simulink model "motion_planner"  (R2015a)
settings: Solver=ode45  StartTime=0.0  StopTime=10.0  RelTol=1e-3
libraries: robotlib x9
settings Model: Creator=Kelan  LastModifiedBy=Kelan

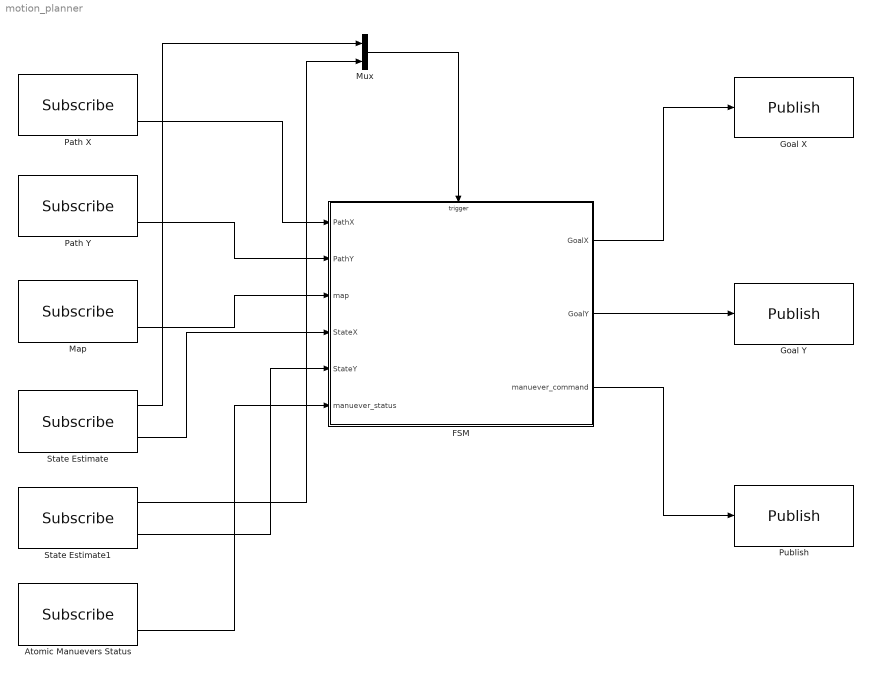
== system motion_planner ==
  Atomic Manuevers Status : robotlib/Subscribe  SourceLibraryInfo=This block requires Robotics System Toolbox  topicSource=Specify your own  topic=/manuevers_status  messageType=std_msgs/Bool  sampleTime=-1  messageQueueLength=1
  FSM : Stateflow chart  TreatAsAtomicUnit=on
  Goal X : robotlib/Publish  SourceLibraryInfo=This block requires Robotics System Toolbox  topicSource=Specify your own  topic=/GoalX  messageType=std_msgs/Int16  messageQueueLength=1
  Goal Y : robotlib/Publish  SourceLibraryInfo=This block requires Robotics System Toolbox  topicSource=Specify your own  topic=/GoalY  messageType=std_msgs/Int16  messageQueueLength=1
  Map : robotlib/Subscribe  SourceLibraryInfo=This block requires Robotics System Toolbox  topicSource=Specify your own  topic=/map  messageType=nav_msgs/OccupancyGrid  sampleTime=-1  messageQueueLength=1
  Mux : Mux  Inputs=2
  Path X : robotlib/Subscribe  SourceLibraryInfo=This block requires Robotics System Toolbox  topicSource=Specify your own  topic=/pathX  messageType=std_msgs/Int16MultiArray  sampleTime=-1  messageQueueLength=1
  Path Y : robotlib/Subscribe  SourceLibraryInfo=This block requires Robotics System Toolbox  topicSource=Specify your own  topic=/pathY  messageType=std_msgs/Int16MultiArray  sampleTime=-1  messageQueueLength=1
  Publish : robotlib/Publish  SourceLibraryInfo=This block requires Robotics System Toolbox  topicSource=Specify your own  topic=/manuever_command  messageType=std_msgs/Char  messageQueueLength=1
  State Estimate : robotlib/Subscribe  SourceLibraryInfo=This block requires Robotics System Toolbox  topicSource=Specify your own  topic=/stateX  messageType=std_msgs/Empty  sampleTime=-1  messageQueueLength=1
  State Estimate1 : robotlib/Subscribe  SourceLibraryInfo=This block requires Robotics System Toolbox  topicSource=Specify your own  topic=/stateY  messageType=std_msgs/Empty  sampleTime=-1  messageQueueLength=1
  wires:
  FSM/1(GoalX) -> Goal X/1
  FSM/2(GoalY) -> Goal Y/1
  FSM/3(manuever_command) -> Publish/1
  Atomic Manuevers Status/2 -> FSM/6(manuever_status)
  State Estimate/2 -> FSM/4(StateX)
  Map/2 -> FSM/3(map)
  Path Y/2 -> FSM/2(PathY)
  Path X/2 -> FSM/1(PathX)
  Mux/1 -> FSM/Trigger
  State Estimate/1 -> Mux/1
  State Estimate1/1 -> Mux/2
  State Estimate1/2 -> FSM/5(StateY)

== stateflow chart motion_planner/FSM ==
  state Initialization
  state Survey [group]
    (junction 123) -> (junction 125) : {loop=0}
    (junction 125) -> (junction 124) [order 1] : [detected=0]
    (junction 124) -> (junction 104) : {GoalY = StateY+10;}
    (junction 105) -> (junction 125) [order 1] : {loop=loop+1}
    (default) -> (junction 125)
    (junction 125) -> (junction 120) [order 2]
    (junction 104) -> (junction 105) : {index=0;}
    (junction 105) -> (junction 111) [order 2] : [(detected=0)&&(index<12)]
    (junction 118) -> (junction 105) : {index=index+1;}
    (junction 111) -> (junction 110) [order 1] : [loop%2=0]
    (junction 111) -> (junction 112) [order 2] : {GoalX = StateX - 10;}
    (junction 110) -> (junction 119) : {GoalX = StateX + 10;}
    (junction 119) -> (junction 112)
    (junction 112) -> (junction 118)
  state Undock
    entry:
    busy=1;
    motion = undock();
  state Scan
    entry:
    busy=1;
    scan=[x,y];
  state Buoy
    entry:
    busy = 1;
    motion = [x, y, r, psi_in, psi_out];
  state Dock
    entry:
    busy=1;
    motion = dock();
  state Hold [group]
    (junction 152) -> (junction 151)
    (junction 151) -> (junction 150) : {GoalX = StateX;
        | GoalY = StateY;
        | manuever_command = 'h'}
    (junction 150) -> (junction 152) : [detected = 0]
  (default) -> Initialization
  Initialization -> (junction 123) : {manuever_status = 1}
  (junction 120) -> (junction 152) : [detected=0]
  data: PathX input; PathY input; map input; StateX input; StateY input; manuever_status input; GoalX output; GoalY output; manuever_command output
  events: detected input RISING_EDGE_EVENT
